simulink model "Logger"  (Simulink 8.8)
settings: Solver=FixedStepAuto  StartTime=0.0  StopTime="Config.SIMULATION_TIME "  FixedStep=0.01  RelTol=1e-3
InitFcn:
  | cd(fileparts(which(bdroot)));
  | initLogger;
undefined symbols (not defined in the file): Config
libraries: WBToolboxLibrary x10
settings Model: SuppressorTable=22 serialization::archive 11 0 3 0 0 0 11 0  Creator=giulio  LastModifiedBy=giulio
settings DataIOCC: LimitDataPoints=off  SaveFormat=Dataset  SignalLoggingSaveFormat=Dataset
settings OptimizationCC: LifeSpan=auto
settings DebuggingCC: UnderspecifiedInitializationDetection=Simplified  MergeDetectMultiDrivingBlocksExec=error  FcnCallInpInsideContextMsg=error  StateNameClashWarn=none  SFUnexpectedBacktrackingDiag=error  SFNoUnconditionalDefaultTransitionDiag=error  SFExecutionAtInitializationDiag=warning
settings HardwareCC: ProdBitPerPointer=64  ProdBitPerSizeT=64  ProdBitPerPtrDiffT=64  ProdLargestAtomicFloat=Float  ProdIntDivRoundTo=Zero  ProdEndianess=LittleEndian  ProdWordSize=64  ProdHWDeviceType=Intel->x86-64 (Windows64)
settings ModelReferenceCC: PropagateSignalLabelsOutOfModel=on
settings GRTTargetCC: TargetLangStandard=C99 (ISO)  GeneratePreprocessorConditionals=Use local settings  CombineOutputUpdateFcns=on  GRTInterface=off
settings ConfigComp: CovMetricSettings=dwe  CovHtmlReporting=off  CovSaveCumulativeToWorkspaceVar=off  CovSaveSingleToWorkspaceVar=off  CovExternalEMLEnable=on

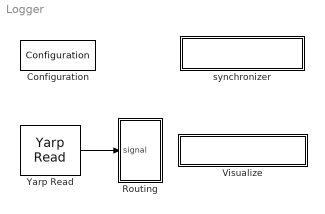
== system Logger ==
  " Visualize" : Subsystem
      mask Display: disp('VISUALIZER')
  Configuration : WBToolboxLibrary/Utilities/Configuration  ConfigSource=Workspace  ConfigObject='WBTConfigRobot'
  "Routing " : Subsystem
  Yarp Read : WBToolboxLibrary/Utilities/Yarp Read  portName='/walking-coordinator/logger/data:o'  signalSize=64  timeout=0.5  blocking=off  timestamp=off  autoconnect=on  errorOnConnection=on
  synchronizer : Subsystem
      mask Display: disp('SYNCHRONIZER')
  wires:
  Yarp Read/1 -> "Routing "/1(signal)

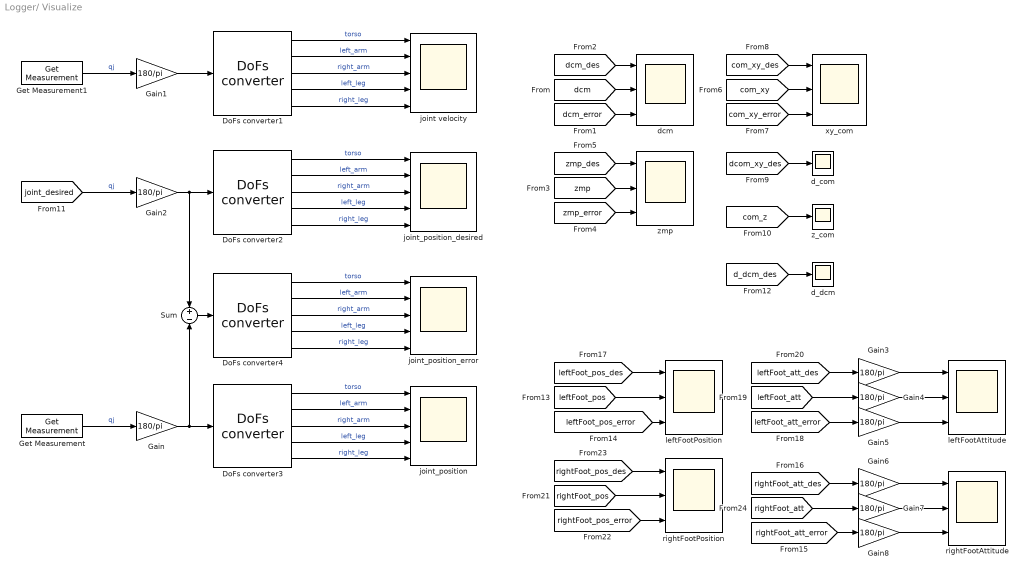
== system Logger/ Visualize ==
  DoFs converter{1..4} (4 alike) : WBToolboxLibrary/Utilities/DoFs converter  yarp2WBIOption=From YARP to WBI
  Gain{,1..8} (9 alike) : Gain  Gain=180/pi
  Get Measurement : WBToolboxLibrary/wholeBodyStates/Get Measurement  measuredType=Joints Position
  Get Measurement1 : WBToolboxLibrary/wholeBodyStates/Get Measurement  measuredType=Joints Velocity
  Sum : Sum  Inputs=+-
  d_com : Scope
  d_dcm : Scope
  "dcm " : Scope  NumInputPorts=3
  joint velocity : Scope  NumInputPorts=5
  "joint_position " : Scope  NumInputPorts=5
  "joint_position_desired " : Scope  NumInputPorts=5
  joint_position_error : Scope  NumInputPorts=5
  leftFootAttitude : Scope  NumInputPorts=3
  leftFootPosition : Scope  NumInputPorts=3
  rightFootAttitude : Scope  NumInputPorts=3
  rightFootPosition : Scope  NumInputPorts=3
  xy_com : Scope  NumInputPorts=3
  z_com : Scope
  zmp : Scope  NumInputPorts=3
  wires:
  [dcom_xy_des] -> d_com/1
  [com_z] -> z_com/1
  [dcm_des] -> "dcm "/1
  [dcm] -> "dcm "/2
  [dcm_error] -> "dcm "/3
  [zmp_des] -> zmp/1
  [zmp_error] -> zmp/3
  [zmp] -> zmp/2
  [com_xy_des] -> xy_com/1
  [com_xy] -> xy_com/2
  [com_xy_error] -> xy_com/3
  Gain/1 -> Sum/2, DoFs converter3/1
  Get Measurement/1 -> Gain/1  "qj"
  DoFs converter3/5 -> "joint_position "/5  "right_leg"
  DoFs converter3/1 -> "joint_position "/1  "torso"
  DoFs converter3/2 -> "joint_position "/2  "left_arm"
  DoFs converter3/4 -> "joint_position "/4  "left_leg"
  DoFs converter3/3 -> "joint_position "/3  "right_arm"
  Gain1/1 -> DoFs converter1/1
  Get Measurement1/1 -> Gain1/1  "qj"
  DoFs converter1/5 -> joint velocity/5  "right_leg"
  DoFs converter1/1 -> joint velocity/1  "torso"
  DoFs converter1/2 -> joint velocity/2  "left_arm"
  DoFs converter1/4 -> joint velocity/4  "left_leg"
  DoFs converter1/3 -> joint velocity/3  "right_arm"
  [joint_desired] -> Gain2/1  "qj"
  Gain2/1 -> Sum/1, DoFs converter2/1
  DoFs converter2/5 -> "joint_position_desired "/5  "right_leg"
  DoFs converter2/1 -> "joint_position_desired "/1  "torso"
  DoFs converter2/2 -> "joint_position_desired "/2  "left_arm"
  DoFs converter2/4 -> "joint_position_desired "/4  "left_leg"
  DoFs converter2/3 -> "joint_position_desired "/3  "right_arm"
  DoFs converter4/5 -> joint_position_error/5  "right_leg"
  DoFs converter4/1 -> joint_position_error/1  "torso"
  DoFs converter4/2 -> joint_position_error/2  "left_arm"
  DoFs converter4/4 -> joint_position_error/4  "left_leg"
  DoFs converter4/3 -> joint_position_error/3  "right_arm"
  Sum/1 -> DoFs converter4/1
  [d_dcm_des] -> d_dcm/1
  [leftFoot_pos_des] -> leftFootPosition/1
  [leftFoot_pos] -> leftFootPosition/2
  [leftFoot_pos_error] -> leftFootPosition/3
  [leftFoot_att] -> Gain4/1
  [leftFoot_att_error] -> Gain5/1
  [leftFoot_att_des] -> Gain3/1
  [rightFoot_pos] -> rightFootPosition/2
  [rightFoot_pos_error] -> rightFootPosition/3
  [rightFoot_pos_des] -> rightFootPosition/1
  [rightFoot_att] -> Gain7/1
  [rightFoot_att_error] -> Gain8/1
  [rightFoot_att_des] -> Gain6/1
  Gain3/1 -> leftFootAttitude/1
  Gain4/1 -> leftFootAttitude/2
  Gain5/1 -> leftFootAttitude/3
  Gain6/1 -> rightFootAttitude/1
  Gain7/1 -> rightFootAttitude/2
  Gain8/1 -> rightFootAttitude/3

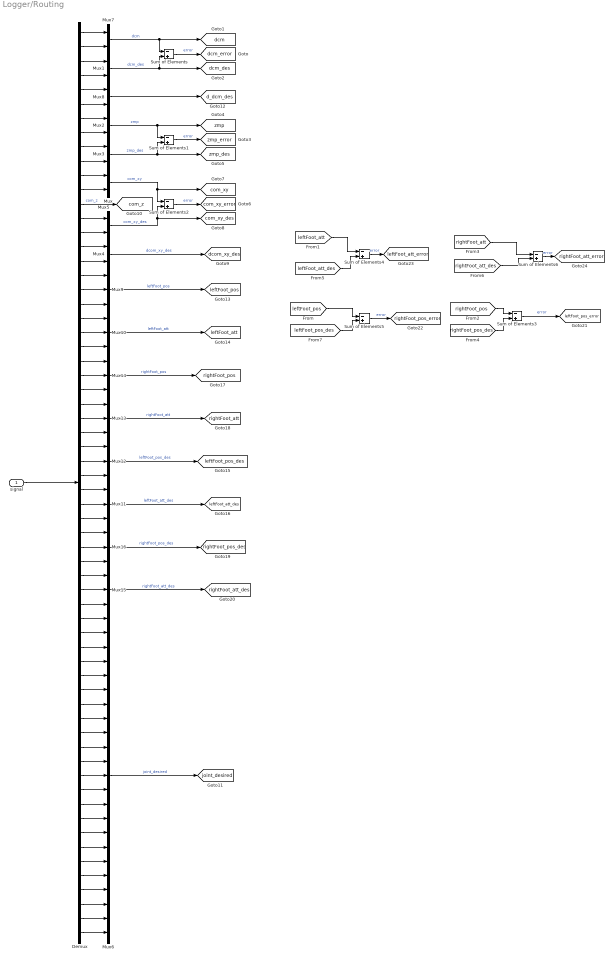
== system Logger/Routing  ==
  signal : Inport
  Demux : Demux  Outputs=64
  Mux{,1..5,7..8} (8 alike) : Mux  Inputs=2
  Mux{9..16} (8 alike) : Mux  Inputs=3
  Mux6 : Mux  Inputs=23
  Sum of Elements{,1..6} (7 alike) : Sum  Inputs=-+
  tag scope: com_xy=global, com_xy_des=global, com_xy_error=global, com_z=global, d_dcm_des=global, dcm=global, dcm_des=global, dcm_error=global, dcom_xy_des=global, joint_desired=global, leftFoot_att=global, leftFoot_att_des=global, leftFoot_att_error=global, leftFoot_pos=global, leftFoot_pos_des=global, leftFoot_pos_error=global, rightFoot_att=global, rightFoot_att_des=global, rightFoot_att_error=global, rightFoot_pos=global, rightFoot_pos_des=global, rightFoot_pos_error=global, zmp=global, zmp_des=global, zmp_error=global
  wires:
  Sum of Elements/1 -> [dcm_error]  "error"
  signal/1 -> Demux/1
  Mux7/1 -> [dcm], Sum of Elements/1  "dcm"
  Mux1/1 -> Sum of Elements/2, [dcm_des]  "dcm_des"
  Mux5/1 -> [com_xy_des], Sum of Elements2/2  "com_xy_des"
  Mux4/1 -> [dcom_xy_des]  "dcom_xy_des"
  Mux/1 -> Sum of Elements2/1, [com_xy]  "com_xy"
  Sum of Elements2/1 -> [com_xy_error]  "error"
  Mux3/1 -> [zmp_des], Sum of Elements1/2  "zmp_des"
  Sum of Elements1/1 -> [zmp_error]  "error"
  Mux2/1 -> [zmp], Sum of Elements1/1  "zmp"
  Mux6/1 -> [joint_desired]  "joint_desired"
  Mux8/1 -> [d_dcm_des]
  Demux/64 -> Mux6/23
  Demux/13 -> [com_z]  "com_z"
  Demux/4 -> Mux1/2
  Demux/5 -> Mux8/1
  Demux/12 -> Mux/2
  Demux/11 -> Mux/1
  Demux/10 -> Mux3/2
  Demux/9 -> Mux3/1
  Demux/8 -> Mux2/2
  Demux/7 -> Mux2/1
  Demux/6 -> Mux8/2
  Demux/14 -> Mux5/1
  Demux/15 -> Mux5/2
  Demux/16 -> Mux4/1
  Demux/17 -> Mux4/2
  Demux/1 -> Mux7/1
  Demux/2 -> Mux7/2
  Demux/3 -> Mux1/1
  Demux/18 -> Mux9/1
  Demux/19 -> Mux9/2
  Demux/20 -> Mux9/3
  Demux/21 -> Mux10/1
  Demux/22 -> Mux10/2
  Demux/23 -> Mux10/3
  Demux/24 -> Mux14/1
  Demux/25 -> Mux14/2
  Demux/26 -> Mux14/3
  Demux/27 -> Mux13/1
  Demux/28 -> Mux13/2
  Demux/29 -> Mux13/3
  Demux/30 -> Mux12/1
  Demux/31 -> Mux12/2
  Demux/32 -> Mux12/3
  Demux/33 -> Mux11/1
  Demux/34 -> Mux11/2
  Demux/35 -> Mux11/3
  Demux/36 -> Mux16/1
  Demux/37 -> Mux16/2
  Demux/38 -> Mux16/3
  Demux/39 -> Mux15/1
  Demux/40 -> Mux15/2
  Demux/41 -> Mux15/3
  Demux/63 -> Mux6/22
  Demux/62 -> Mux6/21
  Demux/61 -> Mux6/20
  Demux/60 -> Mux6/19
  Demux/59 -> Mux6/18
  Demux/58 -> Mux6/17
  Demux/57 -> Mux6/16
  Demux/56 -> Mux6/15
  Demux/55 -> Mux6/14
  Demux/54 -> Mux6/13
  Demux/53 -> Mux6/12
  Demux/52 -> Mux6/11
  Demux/51 -> Mux6/10
  Demux/50 -> Mux6/9
  Demux/49 -> Mux6/8
  Demux/42 -> Mux6/1
  Demux/43 -> Mux6/2
  Demux/44 -> Mux6/3
  Demux/45 -> Mux6/4
  Demux/46 -> Mux6/5
  Demux/47 -> Mux6/6
  Demux/48 -> Mux6/7
  Mux14/1 -> [rightFoot_pos]  "rightFoot_pos"
  Mux9/1 -> [leftFoot_pos]  "leftFoot_pos"
  Mux13/1 -> [rightFoot_att]  "rightFoot_att"
  Mux10/1 -> [leftFoot_att]  "leftFoot_att"
  Mux16/1 -> [rightFoot_pos_des]  "rightFoot_pos_des"
  Mux12/1 -> [leftFoot_pos_des]  "leftFoot_pos_des"
  Mux15/1 -> [rightFoot_att_des]  "rightFoot_att_des"
  Mux11/1 -> [leftFoot_att_des]  "leftFoot_att_des"
  Sum of Elements3/1 -> [leftFoot_pos_error]  "error"
  Sum of Elements5/1 -> [rightFoot_pos_error]  "error"
  Sum of Elements6/1 -> [rightFoot_att_error]  "error"
  Sum of Elements4/1 -> [leftFoot_att_error]  "error"
  [leftFoot_pos] -> Sum of Elements5/1
  [leftFoot_att] -> Sum of Elements4/1
  [rightFoot_att] -> Sum of Elements6/1
  [rightFoot_pos] -> Sum of Elements3/1
  [rightFoot_att_des] -> Sum of Elements6/2
  [leftFoot_att_des] -> Sum of Elements4/2
  [rightFoot_pos_des] -> Sum of Elements3/2
  [leftFoot_pos_des] -> Sum of Elements5/2

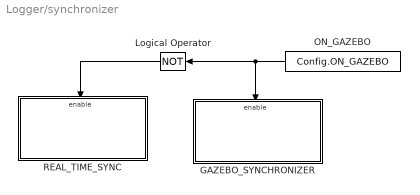
== system Logger/synchronizer ==
  GAZEBO_SYNCHRONIZER : Subsystem
  Logical Operator : Logic  Operator=NOT  AllPortsSameDT=off  OutDataTypeStr=boolean
  "ON_GAZEBO " : Constant  Value=Config.ON_GAZEBO
  REAL_TIME_SYNC : Subsystem
  wires:
  Logical Operator/1 -> REAL_TIME_SYNC/Enable
  "ON_GAZEBO "/1 -> GAZEBO_SYNCHRONIZER/Enable, Logical Operator/1

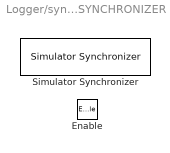
== system Logger/synchronizer/GAZEBO_SYNCHRONIZER ==
  Enable : EnablePort
  Simulator Synchronizer : WBToolboxLibrary/Utilities/Simulator Synchronizer  period=Config.Ts  serverPortName='/clock/rpc'  clientPortName='/WBT_synchronizer/rpc:o'

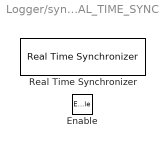
== system Logger/synchronizer/REAL_TIME_SYNC ==
  Enable : EnablePort
  Real Time Synchronizer : WBToolboxLibrary/Utilities/Real Time Synchronizer  period=Config.Ts
